simulink subsystem "rocket"  (R2024b)
settings: Solver=VariableStepAuto  StartTime=0.0  StopTime=10.0  RelTol=1e-3
undefined symbols (not defined in the file or in its folder): GRAVITY, GROUND_LEVEL, MASS_DRY, position_init, velocity_init
libraries: aerolibatmos2 x1
settings Model: Creator=yevge  LastModifiedBy=yevge

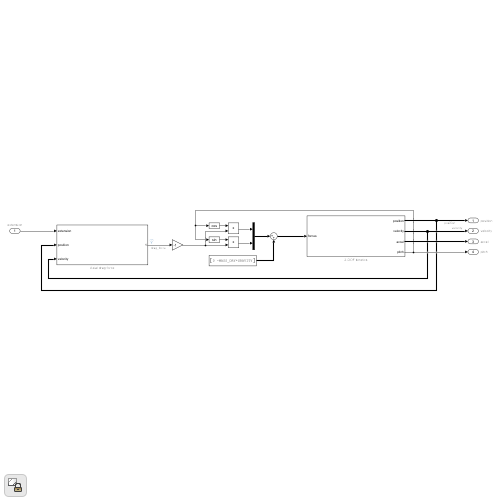
[thumbnail: Simulink's stored preview of the top-level diagram]
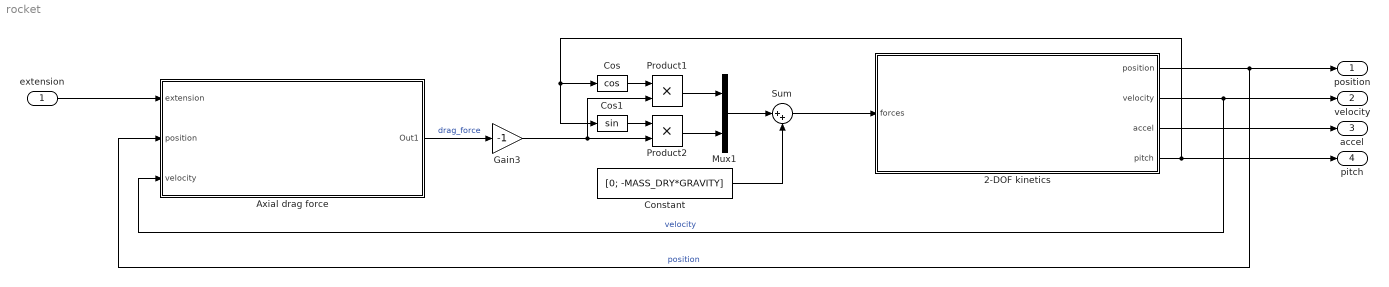
== system rocket ==
  extension : Inport  OutMin=0  OutMax=1  Unit=1  PortDimensions=1
  2-DOF kinetics : Subsystem
  Axial drag force : Subsystem
  Constant : Constant  Value=[0; -MASS_DRY*GRAVITY]
  Cos : Trigonometry  Operator=cos
  Cos1 : Trigonometry
  Gain3 : Gain  Gain=-1
  Mux1 : Mux  Inputs=2
  Product1 : Product
  Product2 : Product
  Sum : Sum  Inputs=|++
  position : Outport  Unit=m  PortDimensions=[2 1]
  velocity : Outport  Port=2  Unit=m/s  PortDimensions=[2 1]
  accel : Outport  Port=3  Unit=m/s^2  PortDimensions=[2 1]
  pitch : Outport  Port=4  Unit=rad  PortDimensions=1
  wires:
  Product1/1 -> Mux1/1
  Constant/1 -> Sum/2
  Sum/1 -> 2-DOF kinetics/1(forces)
  Product2/1 -> Mux1/2
  Gain3/1 -> Product2/2, Product1/2
  Cos1/1 -> Product2/1
  2-DOF kinetics/4(pitch) -> Cos/1, Cos1/1, pitch/1
  Cos/1 -> Product1/1
  Mux1/1 -> Sum/1
  Axial drag force/1(Out1) -> Gain3/1  "drag_force"
  2-DOF kinetics/2(velocity) -> Axial drag force/3(velocity), velocity/1  "velocity"
  2-DOF kinetics/1(position) -> Axial drag force/2(position), position/1  "position"
  2-DOF kinetics/3(accel) -> accel/1
  extension/1 -> Axial drag force/1(extension)

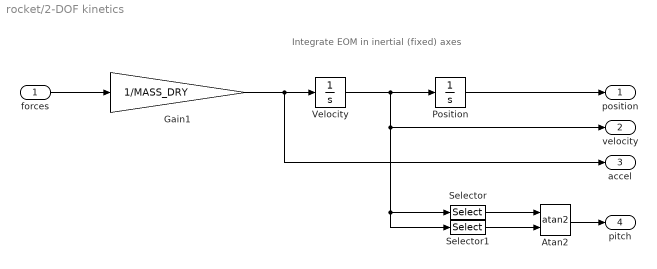
== system rocket/2-DOF kinetics ==
  note: Integrate EOM in inertial (fixed) axes
  forces : Inport  Unit=N  PortDimensions=[2 1]
  Atan2 : Trigonometry  Operator=atan2
  Gain1 : Gain  Gain=1/MASS_DRY
  Position : Integrator  InitialCondition=position_init  ContinuousStateAttributes='position'
  Selector : Selector  InputPortWidth=2  IndexOptions=Index vector (dialog)  Indices=2  OutputSizes=1
  Selector1 : Selector  InputPortWidth=2  IndexOptions=Index vector (dialog)  Indices=1  OutputSizes=1
  Velocity : Integrator  InitialCondition=velocity_init  ContinuousStateAttributes='velocity'
  position : Outport  Unit=m  PortDimensions=[2 1]
  velocity : Outport  Port=2  Unit=m/s  PortDimensions=[2 1]
  accel : Outport  Port=3  Unit=m/s^2  PortDimensions=[2 1]
  pitch : Outport  Port=4  Unit=rad  PortDimensions=1
  wires:
  Atan2/1 -> pitch/1
  Selector1/1 -> Atan2/2
  Selector/1 -> Atan2/1
  Position/1 -> position/1
  forces/1 -> Gain1/1
  Gain1/1 -> Velocity/1, accel/1
  Velocity/1 -> Position/1, velocity/1, Selector/1, Selector1/1

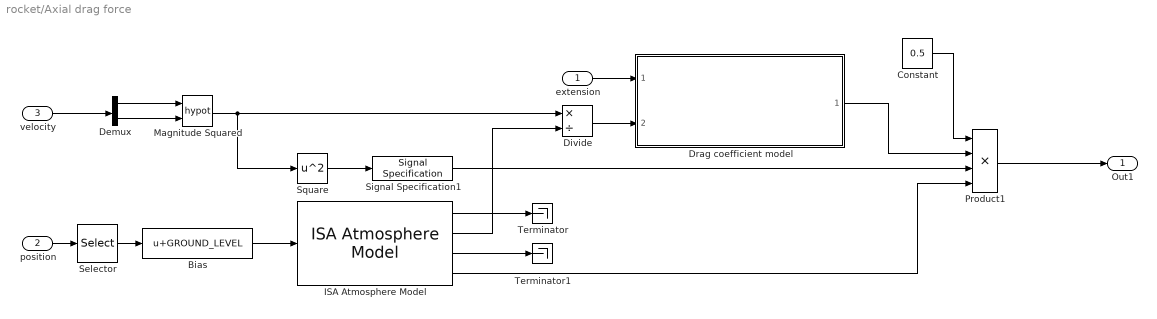
== system rocket/Axial drag force ==
  extension : Inport  OutMin=0  OutMax=1  Unit=1  PortDimensions=1
  position : Inport  Port=2  Unit=m  PortDimensions=[2 1]
  velocity : Inport  Port=3  Unit=m/s  PortDimensions=[2 1]
  Bias : Bias  Bias=GROUND_LEVEL  SaturateOnIntegerOverflow=off
  Constant : Constant  Value=0.5
  Demux : Demux  Outputs=2
  Divide : Product  Inputs=*/
  Drag coefficient model : Subsystem  ReferencedSubsystem=approximate_drag
  ISA Atmosphere Model : aerolibatmos2/ISA Atmosphere Model  useExtended=off  action=Warning  custom=off  viscosityOut=off  g=9.80665  gamma=1.4  R=287.0531  L=0.0065  h_trop=11000  h_strat=20000  rho0=1.225  P0=101325  T0=288.15  h0=0  S=110.4  Tref=273.15  muref=1.716e-5
  Magnitude Squared : Math  Operator=hypot
  Product1 : Product  Inputs=4
  Selector : Selector  InputPortWidth=2  IndexOptions=Index vector (dialog)  Indices=2  OutputSizes=1
  Signal Specification1 : SignalSpecification  Unit=m^2/s^2  Dimensions=1
  Square : Math  Operator=square
  Terminator : Terminator
  Terminator1 : Terminator
  Out1 : Outport  Unit=N  PortDimensions=1
  wires:
  Divide/1 -> Drag coefficient model/2
  extension/1 -> Drag coefficient model/1
  Signal Specification1/1 -> Product1/3
  Drag coefficient model/1 -> Product1/2
  Constant/1 -> Product1/1
  Square/1 -> Signal Specification1/1
  ISA Atmosphere Model/4 -> Product1/4
  ISA Atmosphere Model/3 -> Terminator1/1
  ISA Atmosphere Model/1 -> Terminator/1
  ISA Atmosphere Model/2 -> Divide/2
  Magnitude Squared/1 -> Divide/1, Square/1
  Demux/2 -> Magnitude Squared/2
  Demux/1 -> Magnitude Squared/1
  Bias/1 -> ISA Atmosphere Model/1
  Selector/1 -> Bias/1
  Product1/1 -> Out1/1
  position/1 -> Selector/1
  velocity/1 -> Demux/1
